simulink model "LCK_old"  (R2018b)
settings: Solver=FixedStepDiscrete  StartTime=0.0  StopTime=inf  FixedStep=0.005  RelTol=1e-3
PostLoadFcn:
  | if any(exist('dsrtsu_mdlpostloadfcn', 'file') ~= 0), dsrtsu_mdlpostloadfcn('Execute', bdroot); end
values from neighbouring files (symbols this model uses):
  C_DEG2RAD = 0.0175    [LCK_Macro.sldd]
  C_KPH2MPS = 0.2778    [LCK_Macro.sldd]
  C_NEARZERO = 0.0001    [LCK_Macro.sldd]
  C_ONE = 1.0    [LCK_Macro.sldd]
  C_RAD2DEG = 57.2958    [LCK_Macro.sldd]
  C_ZERO = 0.0    [LCK_Macro.sldd]
  k_accel_pedal_pos_per_speed_x : value not decoded    [LCK_LogicPara.sldd]
  k_accel_pedal_pos_per_speed_z : value not decoded    [LCK_LogicPara.sldd]
  k_brake_suprress_hold = 1000.0    [LCK_LogicPara.sldd]
  k_driver_appl_torque_filt = 50.0    [LCK_LogicPara.sldd]
  k_driver_suppression_hold_time = 3000.0    [LCK_LogicPara.sldd]
  k_hands_on_wheel_hold_msec = 500.0    [LCK_LogicPara.sldd]
  k_hands_on_wheel_torque_hi = 0.2    [LCK_LogicPara.sldd]
  k_hands_on_wheel_torque_lo = 0.15    [LCK_LogicPara.sldd]
  k_handsoff_delay_cycles = 50.0    [LCK_LogicPara.sldd]
  k_handsoff_torq_Lo_CR = 0.3    [LCK_LogicPara.sldd]
  k_handson_delay_cycles = 5.0    [LCK_LogicPara.sldd]
  k_HighAccel_suppress_hold = 3000.0    [LCK_LogicPara.sldd]
  k_HLR_suprress_hold = 3000.0    [LCK_LogicPara.sldd]
  k_hs_StrAng_CR_threshold_z : value not decoded    [LCK_LogicPara.sldd]
  k_LC_Exit_Switch = 0.0    [LCK_LogicPara.sldd]
  k_LCG_Configured = 1.0    [LCK_LogicPara.sldd]
  k_LCK_A0_Rdy2Act_UseConst = 0.0    [LCK_LogicPara.sldd]
  k_LCK_A0Fac_ActSta : value not decoded    [LCK_CtrlPara.sldd]
  k_LCK_A0Fac_DrvStm : value not decoded    [LCK_CtrlPara.sldd]
  k_LCK_A0Shift_LftCurv : value not decoded    [LCK_CtrlPara.sldd]
  k_LCK_A0Shift_RgtCurv : value not decoded    [LCK_CtrlPara.sldd]
  k_LCK_A0Shift_StraLan = 0.0    [LCK_CtrlPara.sldd]
  k_LCK_A0ShiftFac_Dy_LftCurv : value not decoded    [LCK_CtrlPara.sldd]
  k_LCK_A0ShiftFac_Dy_RgtCurv : value not decoded    [LCK_CtrlPara.sldd]
  k_LCK_A0ShiftFac_Vspd : value not decoded    [LCK_CtrlPara.sldd]
  k_LCK_accel_inhibit_thold = 35.0    [LCK_LogicPara.sldd]
  k_LCK_Active2Ready_Mask = 255.0    [LCK_LogicPara.sldd]
  k_LCK_CvatRateBks : value not decoded    [LCK_CtrlPara.sldd]
  k_LCK_CvatrBks : value not decoded    [LCK_CtrlPara.sldd]
  k_LCK_DFac_Dy : value not decoded    [LCK_CtrlPara.sldd]
  k_LCK_DFac_Dy_Curv : value not decoded    [LCK_CtrlPara.sldd]
  k_LCK_DFac_HaCurCen : value not decoded    [LCK_CtrlPara.sldd]
  k_LCK_DFac_HaCurSid : value not decoded    [LCK_CtrlPara.sldd]
  k_LCK_DFac_HadCurCen : value not decoded    [LCK_CtrlPara.sldd]
  k_LCK_DFac_HadCurSid : value not decoded    [LCK_CtrlPara.sldd]
  k_LCK_DFac_HadStrCen : value not decoded    [LCK_CtrlPara.sldd]
  k_LCK_DFac_HadStrSid : value not decoded    [LCK_CtrlPara.sldd]
  k_LCK_DFac_HaStrCen : value not decoded    [LCK_CtrlPara.sldd]
  k_LCK_DFac_HaStrSid : value not decoded    [LCK_CtrlPara.sldd]
  k_LCK_DFac_Rad : value not decoded    [LCK_CtrlPara.sldd]
  k_LCK_DFac_SA_CurCen : value not decoded    [LCK_CtrlPara.sldd]
  k_LCK_DFac_SA_CurSid : value not decoded    [LCK_CtrlPara.sldd]
  k_LCK_DFac_SA_StrCen : value not decoded    [LCK_CtrlPara.sldd]
  k_LCK_DFac_SA_StrSid : value not decoded    [LCK_CtrlPara.sldd]
  k_LCK_DFac_SS_CurCen : value not decoded    [LCK_CtrlPara.sldd]
  k_LCK_DFac_SS_CurSid : value not decoded    [LCK_CtrlPara.sldd]
  k_LCK_DFac_SS_StrCen : value not decoded    [LCK_CtrlPara.sldd]
  k_LCK_DFac_SS_StrSid : value not decoded    [LCK_CtrlPara.sldd]
  k_LCK_DFac_Vspd : value not decoded    [LCK_CtrlPara.sldd]
  k_LCK_DlyTm_DrvStim = 0.2    [LCK_CtrlPara.sldd]
  k_LCK_DTermMax = 2.0    [LCK_CtrlPara.sldd]
  k_LCK_DyBks_Curv : value not decoded    [LCK_CtrlPara.sldd]
  k_LCK_Enable_POOnly = 1.0    [LCK_LogicPara.sldd]
  k_LCK_Entry_DistBuffer = 0.1    [LCK_LogicPara.sldd]
  k_LCK_Fac_Vspd2RngThr_FalRec = 0.23    [LCK_CtrlPara.sldd]
  k_LCK_Ffw_CvatSwh = 0.0    [LCK_CtrlPara.sldd]
  k_LCK_Ffw_DyBks : value not decoded    [LCK_CtrlPara.sldd]
  k_LCK_Ffw_TimCon_CmdFlt = 0.0    [LCK_CtrlPara.sldd]
  k_LCK_FfwDeltaFac_Rad_Lft : value not decoded    [LCK_CtrlPara.sldd]
  k_LCK_FfwDeltaFac_Rad_Rgt : value not decoded    [LCK_CtrlPara.sldd]
  k_LCK_FfwDeltaFac_Vspd : value not decoded    [LCK_CtrlPara.sldd]
  k_LCK_FfwFac_CvatRate_Lft : value not decoded    [LCK_CtrlPara.sldd]
  k_LCK_FfwFac_CvatRate_Rgt : value not decoded    [LCK_CtrlPara.sldd]
  k_LCK_FfwFac_Dy : value not decoded    [LCK_CtrlPara.sldd]
  k_LCK_FfwFac_Rad_Lft : value not decoded    [LCK_CtrlPara.sldd]
  k_LCK_FfwFac_Rad_Rgt : value not decoded    [LCK_CtrlPara.sldd]
  k_LCK_FfwFac_Vspd : value not decoded    [LCK_CtrlPara.sldd]
  k_LCK_FfwTorq_Cvat : value not decoded    [LCK_CtrlPara.sldd]
  k_LCK_HAFac_ActSta : value not decoded    [LCK_CtrlPara.sldd]
  k_LCK_HAFac_DrvStm : value not decoded    [LCK_CtrlPara.sldd]
  k_LCK_HaloTime = 2000.0    [LCK_LogicPara.sldd]
  k_LCK_HaloTime_Switch = 0.0    [LCK_LogicPara.sldd]
  k_LCK_HARFac_ActSta : value not decoded    [LCK_CtrlPara.sldd]
  k_LCK_HARFac_DrvStm : value not decoded    [LCK_CtrlPara.sldd]
  k_LCK_Hed_DyBks : value not decoded    [LCK_CtrlPara.sldd]
  k_LCK_HedAngDiffX : value not decoded    [LCK_CtrlPara.sldd]
  k_LCK_HedAngRateDiffX : value not decoded    [LCK_CtrlPara.sldd]
  k_LCK_HndsOnWhel_DlyTm_Idl2Rdy = 0.0    [LCK_LogicPara.sldd]
  k_LCK_host_veh_width = 1.86    [LCK_LogicPara.sldd]
  k_LCK_Idle2Ready_Mask = 239.0    [LCK_LogicPara.sldd]
  k_LCK_Junc_SusTime = 1.0    [LCK_LogicPara.sldd]
  k_LCK_KpKdDecSlopeLmt = 10.0    [LCK_CtrlPara.sldd]
  k_LCK_KpKdIncSlopeLmt = 5.0    [LCK_CtrlPara.sldd]
  k_LCK_Lat_Ctrl_DFac_Lft = 1.0    [LCK_CtrlPara.sldd]
  k_LCK_Lat_Ctrl_DFac_Rgt = 1.05    [LCK_CtrlPara.sldd]
  k_LCK_Lat_Ctrl_Kd = 0.8    [LCK_CtrlPara.sldd]
  k_LCK_Lat_Ctrl_Ki = 0.5    [LCK_CtrlPara.sldd]
  k_LCK_Lat_Ctrl_Kp = 0.7    [LCK_CtrlPara.sldd]
  k_LCK_Lat_Ctrl_Kp_NearGain = 0.7    [LCK_CtrlPara.sldd]
  k_LCK_Lat_Ctrl_PFac_Lft = 1.0    [LCK_CtrlPara.sldd]
  k_LCK_Lat_Ctrl_PFac_Rgt = 1.05    [LCK_CtrlPara.sldd]
  k_LCK_Lat_Ctrl_TimCon_CmdFlt = 5.0    [LCK_CtrlPara.sldd]
  k_LCK_Lat_DFac_Rad : value not decoded    [LCK_CtrlPara.sldd]
  k_LCK_Lat_DFac_SS_Cur : value not decoded    [LCK_CtrlPara.sldd]
  k_LCK_Lat_DFac_SS_Str : value not decoded    [LCK_CtrlPara.sldd]
  k_LCK_Lat_DFac_Vspd : value not decoded    [LCK_CtrlPara.sldd]
  k_LCK_Lat_DyBks : value not decoded    [LCK_CtrlPara.sldd]
  k_LCK_Lat_IFac_Rad : value not decoded    [LCK_CtrlPara.sldd]
  k_LCK_Lat_IFac_Vspd : value not decoded    [LCK_CtrlPara.sldd]
  k_LCK_Lat_ILmtFac_Dy_CurvLan : value not decoded    [LCK_CtrlPara.sldd]
  k_LCK_Lat_ILmtFac_Dy_StraLan : value not decoded    [LCK_CtrlPara.sldd]
  k_LCK_Lat_ILmtFac_Rad : value not decoded    [LCK_CtrlPara.sldd]
  k_LCK_Lat_ILmtFac_Rad_NearGain = 1.0    [LCK_CtrlPara.sldd]
  k_LCK_Lat_ILmtFac_Vspd_CurvLan : value not decoded    [LCK_CtrlPara.sldd]
  k_LCK_Lat_ILmtFac_Vspd_StraLan : value not decoded    [LCK_CtrlPara.sldd]
  k_LCK_Lat_ITermLmt_Dy = 1.0    [LCK_CtrlPara.sldd]
  k_LCK_Lat_KpKdDecSlopeLmt = 10.0    [LCK_CtrlPara.sldd]
  k_LCK_Lat_KpKdIncSlopeLmt = 10.0    [LCK_CtrlPara.sldd]
  k_LCK_Lat_PFac_Dy_InnLftCur : value not decoded    [LCK_CtrlPara.sldd]
  k_LCK_Lat_PFac_Dy_InnRgtCur : value not decoded    [LCK_CtrlPara.sldd]
  k_LCK_Lat_PFac_Dy_OutLftCur : value not decoded    [LCK_CtrlPara.sldd]
  k_LCK_Lat_PFac_Dy_OutRgtCur : value not decoded    [LCK_CtrlPara.sldd]
  k_LCK_Lat_PFac_Dy_Str : value not decoded    [LCK_CtrlPara.sldd]
  k_LCK_Lat_PFac_Rad : value not decoded    [LCK_CtrlPara.sldd]
  ... (+158 more)
undefined symbols (not defined in the file or in its folder): k_LCK_CurvBks, K_LCK_SPA0A1A2_LMRngCmp_y
libraries: LateralControl_fcns_lib x58, simulink x22
(part 29 of 45)

== system LCK_old/Lateral_Control_Module/LCK_State_Ctrl/LCK_Mode_Transition/Determination_of_READY2OFF ==
  TJA_Switch : Inport
  LCK_Switch : Inport  Port=2
  Logical Operator3 : Logic  Tag={'date',737184.60397805553}  Description=_GWMAB30P2.LCK.000_1110_  Operator=NOR  AllPortsSameDT=off  OutDataTypeStr=boolean
  READY2OFF : Outport
  wires:
  TJA_Switch/1 -> Logical Operator3/1
  LCK_Switch/1 -> Logical Operator3/2
  Logical Operator3/1 -> READY2OFF/1

== system LCK_old/Lateral_Control_Module/LCK_State_Ctrl/LCK_Mode_Transition/Determination_of_SPP_Valid ==
  note: 0x0: Invalid
      | 0x1: LLM_Only
      | 0x2: RLM_Only
      | 0x3: BLM_Only
      | 0x4: PO_Only
      | 0x5: PO_and_LLM
      | 0x6: PO_and_RLM
      | 0x7: PO_and_BLM
      | 0x8: Reserved
  SP_type : Inport
  SP_conf : Inport  Port=2
  Constant4 : Constant  Tag={'output',{'name','$P','class','EXTERN_MACRO','type','UInt8'},'date',737531.63293407403}  Description=_GACA26P4.LCK.000_11_  Value=TJA_SP_TYPE_POONLY
  Constant48 : Constant  Tag={'output',{'name','$P','class','EXTERN_MACRO','type','UInt8'},'date',737503.54713141208}  Description=_GACA26P3.LCK.000_6_  Value=TJA_SP_CONF_MEDIUM
  Constant49 : Constant  Tag={'output',{'name','$P','class','EXTERN_MACRO','type','UInt8'},'date',737237.80253754626}  Description=_GWMAB30P3.LCK.000_45_  Value=TJA_SP_TYPE_BLMONLY
  Constant60 : Constant  Tag={'output',{'name','$P','class','EXTERN_MACRO','type','UInt8'},'date',737237.80260364583}  Description=_GWMAB30P3.LCK.000_55_  Value=TJA_SP_TYPE_POBLM
  Constant7 : Constant  Tag={'output',{'name','$P','class','EXTERN_CAL','type','Bool'},'date',737531.63312886574}  Description=_GACA26P4.LCK.000_12_  Value=k_LCK_Enable_POOnly
  Data Type Conversion23 : DataTypeConversion  Description=_GWMAB30P4.LCK.000_134_
  Data Type Conversion24 : DataTypeConversion  Description=_GWMAB30P4.LCK.000_135_
  Logical Operator150 : Logic  Tag={'date',737531.60590518522}  Description=_GACA26P4.LCK.000_30_  Operator=OR  AllPortsSameDT=off  OutDataTypeStr=boolean
  Logical Operator50 : Logic  Tag={'date',737237.63746805559}  Description=_GWMAB30P3.LCK.000_68_  Inputs=4  AllPortsSameDT=off  OutDataTypeStr=boolean
  Logical Operator51 : Logic  Tag={'date',737237.63746818283}  Description=_GWMAB30P3.LCK.000_69_  AllPortsSameDT=off  OutDataTypeStr=boolean
  Logical Operator53 : Logic  Tag={'date',737237.63746843755}  Description=_GWMAB30P3.LCK.000_71_  Operator=OR  AllPortsSameDT=off  OutDataTypeStr=boolean
  Relational Operator202 : RelationalOperator  Tag={'date',737531.60601208336}  Description=_GACA26P4.LCK.000_36_  Operator=~=  OutDataTypeStr=boolean  RndMeth=Nearest
  Relational Operator24 : RelationalOperator  Tag={'date',737237.63747119217}  Description=_GWMAB30P3.LCK.000_87_  Operator=<=  OutDataTypeStr=boolean  RndMeth=Nearest
  Relational Operator25 : RelationalOperator  Tag={'date',737237.63747133105}  Description=_GWMAB30P3.LCK.000_88_  Operator=>  OutDataTypeStr=boolean  RndMeth=Nearest
  Relational Operator28 : RelationalOperator  Tag={'date',737237.63747158565}  Description=_GWMAB30P3.LCK.000_90_  Operator===  OutDataTypeStr=boolean  RndMeth=Nearest
  Relational Operator43 : RelationalOperator  Tag={'date',737237.63747218752}  Description=_GWMAB30P3.LCK.000_93_  OutDataTypeStr=boolean  RndMeth=Nearest
  Relational Operator50 : RelationalOperator  Tag={'date',737237.63747292827}  Description=_GWMAB30P3.LCK.000_98_  Operator===  OutDataTypeStr=boolean  RndMeth=Nearest
  k_LCK_SPTyp_LowLmt_Idl2Rdy1 : Constant  Tag={'output',{'name','$P','class','EXTERN_CAL','type','UInt8'},'date',737246.86453388887}  Description=_GWMAB30P3.LCK.000_137_  Value=k_LCK_SPTyp_LowLmt_Idl2Rdy
  k_LCK_SPTyp_UpLmt_Idl2Rdy1 : Constant  Tag={'output',{'name','$P','class','EXTERN_CAL','type','UInt8'},'date',737246.86453350692}  Description=_GWMAB30P3.LCK.000_139_  Value=k_LCK_SPTyp_UpLmt_Idl2Rdy
  SP_valid_low_spd : Outport
  SP_valid_high_spd : Outport  Port=2
  wires:
  Relational Operator25/1 -> Logical Operator50/4, Logical Operator51/1
  SP_type/1 -> [SP_type], Relational Operator24/1, Relational Operator43/1, Relational Operator202/1
  Data Type Conversion24/1 -> SP_valid_low_spd/1
  Relational Operator50/1 -> Logical Operator53/2
  Logical Operator53/1 -> Logical Operator51/2
  Relational Operator43/1 -> Logical Operator50/3
  Logical Operator50/1 -> Data Type Conversion24/1
  [SP_type] -> Relational Operator28/2, Relational Operator50/1
  Constant60/1 -> Relational Operator50/2
  Constant7/1 -> Logical Operator150/2
  k_LCK_SPTyp_LowLmt_Idl2Rdy1/1 -> Relational Operator43/2
  Constant4/1 -> Relational Operator202/2
  Relational Operator28/1 -> Logical Operator53/1
  Logical Operator51/1 -> Data Type Conversion23/1
  Relational Operator202/1 -> Logical Operator150/1
  Logical Operator150/1 -> Logical Operator50/1
  Constant49/1 -> Relational Operator28/1
  k_LCK_SPTyp_UpLmt_Idl2Rdy1/1 -> Relational Operator24/2
  Relational Operator24/1 -> Logical Operator50/2
  Constant48/1 -> Relational Operator25/2
  SP_conf/1 -> Relational Operator25/1
  Data Type Conversion23/1 -> SP_valid_high_spd/1

== system LCK_old/Lateral_Control_Module/LCK_State_Ctrl/LCK_Mode_Transition/Determination_of_Short_LM_Range ==
  VIS_LANE_LEFT_INDIVID_RANGE : Inport
  VIS_LANE_RIGHT_INDIVID_RANGE : Inport  Port=2
  veh_speed_kph : Inport  Port=3
  Data Type Conversion95 : DataTypeConversion
  Delay_Trig : LateralControl_fcns_lib/Delay_Trig  SystemSampleTime=-1
  Logical Operator159 : Logic  Inputs=3  AllPortsSameDT=off  OutDataTypeStr=boolean
  Product : Product
  Relational Operator213 : RelationalOperator  Operator=<=  OutDataTypeStr=boolean  RndMeth=Nearest
  Relational Operator216 : RelationalOperator  OutDataTypeStr=boolean  RndMeth=Nearest
  Relational Operator217 : RelationalOperator  OutDataTypeStr=boolean  RndMeth=Nearest
  k_LCK_LowRng_Spd_Thr : Constant  Value=k_LCK_LowRng_Spd_Thr
  k_LCK_Rng2VehSpd_Ratio_DlyTime : Constant  Value=k_LCK_Rng2VehSpd_Ratio_DlyTime
  k_LCK_Rng2VehSpd_Ratio_Thr : Constant  Value=k_LCK_Rng2VehSpd_Ratio_Thr
  Short_LM_Range : Outport
  wires:
  [veh_speed_kph] -> Relational Operator217/1
  Product/1 -> Relational Operator213/2, Relational Operator216/1
  Logical Operator159/1 -> Data Type Conversion95/1
  k_LCK_Rng2VehSpd_Ratio_DlyTime/1 -> Delay_Trig/2
  Relational Operator213/1 -> Logical Operator159/1
  Relational Operator216/1 -> Logical Operator159/2
  Relational Operator217/1 -> Logical Operator159/3
  k_LCK_Rng2VehSpd_Ratio_Thr/1 -> Product/2
  Data Type Conversion95/1 -> Delay_Trig/1
  k_LCK_LowRng_Spd_Thr/1 -> Relational Operator217/2
  VIS_LANE_RIGHT_INDIVID_RANGE/1 -> Relational Operator216/2
  veh_speed_kph/1 -> [veh_speed_kph], Product/1
  VIS_LANE_LEFT_INDIVID_RANGE/1 -> Relational Operator213/1
  Delay_Trig/1 -> Short_LM_Range/1

== system LCK_old/Lateral_Control_Module/LCK_State_Ctrl/LCK_Mode_Transition/Determination_of_TJA_Switch ==
  TJA_Switch_Input : Inport
  Constant19 : Constant  Tag={'output',{'type','Int32'},'date',737184.60397266201}  Description=_GWMAB30P2.LCK.000_1069_  Value=0
  Switch5 : Switch  Tag={'output',{'type','Bool'},'threshold',{'type','Int32'},'date',737189.64659098384}  Description=_GWMAB30P2.LCK.000_1195_  Threshold=0.5
  k_LCK_VisionOnly : Constant  Tag={'output',{'name','$P','class','EXTERN_CAL','type','Bool'},'date',737246.86429052078}  Description=_GWMAB30P2.LCK.000_1268_  Value=k_LCK_VisionOnly
  TJA_Switch : Outport
  wires:
  Switch5/1 -> TJA_Switch/1
  Constant19/1 -> Switch5/1
  k_LCK_VisionOnly/1 -> Switch5/2, [LCK_VisionOnly]
  TJA_Switch_Input/1 -> Switch5/3
